simulink model "aerodynamic_model"  (R2021a)
settings: Solver=FixedStepAuto  StartTime=0  StopTime=10.0  FixedStep=T_sample_control  RelTol=1e-3  EnableMultiTasking=on
model workspace (MAT data in the model file):
  wing_alpha = 0.785398163397
libraries: vrlib x2
settings Model: DataDictionary=pid.sldd  EnableAccessToBaseWorkspace=off  ModifiedByFormat=The MathWorks Inc.  Creator=The MathWorks, Inc.  LastModifiedBy=The MathWorks Inc.
settings SolverCC: AlgebraicLoopSolver=TrustRegion
settings DataIOCC: SaveFormat=StructureWithTime  ReturnWorkspaceOutputs=off
settings OptimizationCC: BlockReduction=off  DefaultParameterBehavior=Inlined  InlineInvariantSignals=on  BufferReuse=off  PassReuseOutputArgsAs=Individual arguments  ExpressionDepthLimit=2147483647  ZeroExternalMemoryAtStartup=off  ZeroInternalMemoryAtStartup=off  EfficientFloat2IntCast=on  LifeSpan=1  EfficientTunableParamExpr=on
settings DebuggingCC: AlgebraicLoopMsg=none  FcnCallInpInsideContextMsg=warning  UnconnectedInputMsg=none  UnconnectedOutputMsg=none  UnconnectedLineMsg=none  UniqueDataStoreMsg=error  AssertControl=DisableAll  AllowSymbolicDim=off  StateNameClashWarn=warning  StrictBusMsg=ErrorOnBusTreatedAsVector  SFUnexpectedBacktrackingDiag=warning  SFNoUnconditionalDefaultTransitionDiag=warning  SFExecutionAtInitializationDiag=none  SFMachineParentedDataDiag=warning  ArithmeticOperatorsInVariantConditions=warning
settings HardwareCC: ProdBitPerPointer=32  ProdBitPerSizeT=32  ProdBitPerPtrDiffT=32  ProdLargestAtomicFloat=None  ProdIntDivRoundTo=Undefined  ProdEndianess=Unspecified  ProdWordSize=32  ProdHWDeviceType=32-bit Generic
settings ModelReferenceCC: PropagateSignalLabelsOutOfModel=off
settings SFSimCC: SimUseLocalCustomCode=off  CustomCodeUndefinedFunction=UseInterfaceOnly
settings RTWCC: SystemTargetFile=ert.tlc  TemplateMakefile=ert_default_tmf  GenerateReport=on  RTWUseLocalCustomCode=off  IncludeHyperlinkInReport=on  GenerateTraceInfo=on  GenerateTraceReport=on  GenerateTraceReportSl=on  GenerateTraceReportSf=on  GenerateTraceReportEml=on  GenerateCodeMetricsReport=on
settings CodeAppCC: IgnoreCustomStorageClasses=off  IgnoreTestpoints=on  CustomSymbolStrType=$N$R$M  StateflowObjectComments=on  InternalIdentifier=Classic
settings ERTTargetCC: MultiwordLength=2048  GenerateSampleERTMain=on  SupportNonFinite=off  ParenthesesLevel=Maximum  InlinedParameterPlacement=NonHierarchical  ERTCustomFileTemplate=example_file_process.tlc  ConvertIfToSwitch=off  SuppressUnreachableDefaultCases=off
settings ConfigComp: CovMetricSettings=dw  CovSaveCumulativeToWorkspaceVar=on  CovSaveSingleToWorkspaceVar=on  CovExternalEMLEnable=off  CovSFcnEnable=off

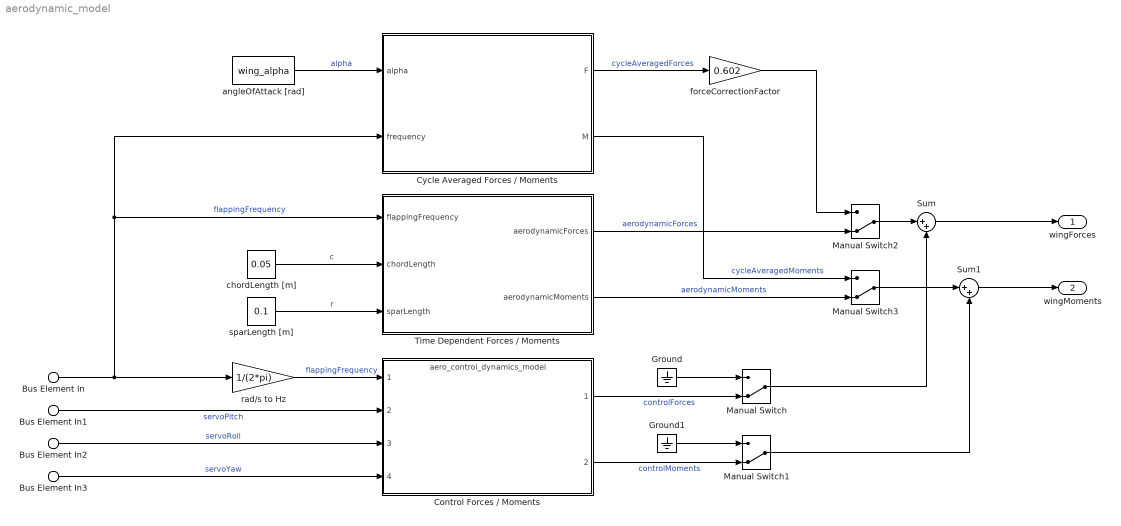
== system aerodynamic_model ==
  Bus Element In : Inport  PortName=flapFreq  Element=flapping_freq
  Bus Element In1 : Inport  PortName=flapFreq  Element=pitch
  Bus Element In2 : Inport  PortName=flapFreq  Element=roll
  Bus Element In3 : Inport  PortName=flapFreq  Element=yaw
  Control Forces / Moments : ModelReference  ModelNameDialog=aero_control_dynamics_model.slx  SimulationMode=Normal  ModelReferenceVersion=1.12
      mask Display: disp('Control Forces and Moments');
  Cycle Averaged Forces / Moments : MATLAB Function  TreatAsAtomicUnit=on
  Ground : Ground
  Ground1 : Ground
  Manual Switch{,1..3} (4 alike) : ManualSwitch  CurrentSetting=0
  Sum : Sum  Inputs=|++
  Sum1 : Sum  Inputs=|++
  Time Dependent Forces / Moments : Subsystem
      mask Display: disp('Time Dependent Forces and Moments');
  angleOfAttack [rad] : Constant  Value=wing_alpha
  chordLength [m] : Constant  Value=0.05
  forceCorrectionFactor : Gain  Gain=0.602
  rad/s to Hz : Gain  Gain=1/(2*pi)
  sparLength [m] : Constant  Value=0.1
  wingForces : Outport  PortDimensions=3
  wingMoments : Outport  Port=2  PortDimensions=3
  wires:
  Bus Element In1/1 -> Control Forces / Moments/2  "servoPitch"
  Bus Element In2/1 -> Control Forces / Moments/3  "servoRoll"
  Bus Element In3/1 -> Control Forces / Moments/4  "servoYaw"
  rad/s to Hz/1 -> Control Forces / Moments/1  "flappingFrequency"
  Sum/1 -> wingForces/1
  Sum1/1 -> wingMoments/1
  Control Forces / Moments/1 -> Manual Switch/2  "controlForces"
  Manual Switch/1 -> Sum/2
  Ground/1 -> Manual Switch/1
  Control Forces / Moments/2 -> Manual Switch1/2  "controlMoments"
  Ground1/1 -> Manual Switch1/1
  Manual Switch1/1 -> Sum1/2
  Bus Element In/1 -> Time Dependent Forces / Moments/1(flappingFrequency), Cycle Averaged Forces / Moments/2(frequency), rad/s to Hz/1  "flappingFrequency"
  angleOfAttack [rad]/1 -> Cycle Averaged Forces / Moments/1(alpha)  "alpha"
  Manual Switch2/1 -> Sum/1
  Cycle Averaged Forces / Moments/1(F) -> forceCorrectionFactor/1  "cycleAveragedForces"
  Manual Switch3/1 -> Sum1/1
  Cycle Averaged Forces / Moments/2(M) -> Manual Switch3/1  "cycleAveragedMoments"
  forceCorrectionFactor/1 -> Manual Switch2/1
  chordLength [m]/1 -> Time Dependent Forces / Moments/2(chordLength)  "c"
  sparLength [m]/1 -> Time Dependent Forces / Moments/3(sparLength)  "r"
  Time Dependent Forces / Moments/1(aerodynamicForces) -> Manual Switch2/2  "aerodynamicForces"
  Time Dependent Forces / Moments/2(aerodynamicMoments) -> Manual Switch3/2  "aerodynamicMoments"

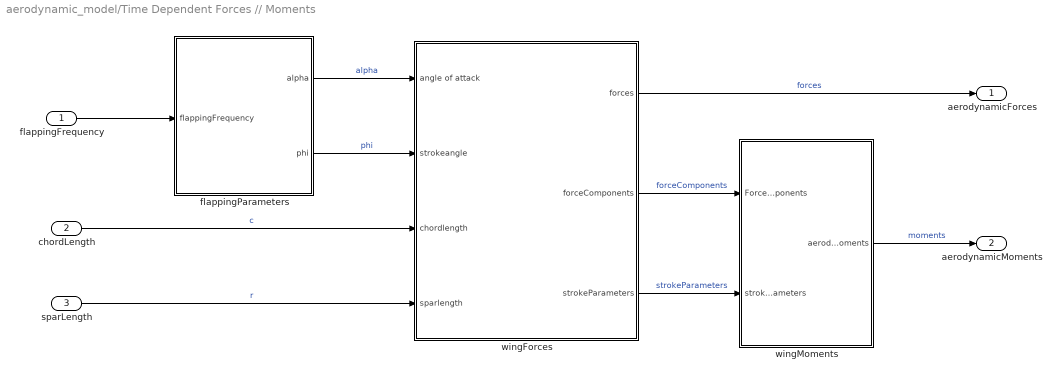
== system aerodynamic_model/Time Dependent Forces // Moments ==
  flappingFrequency : Inport
  chordLength : Inport  Port=2
  sparLength : Inport  Port=3
  flappingParameters : Subsystem
      mask Display: disp('Flapping Parameters');
  wingForces : Subsystem
      mask Display: disp('Wing Forces');
  wingMoments : Subsystem
      mask Display: disp('Wing Moments');
  aerodynamicForces : Outport
  aerodynamicMoments : Outport  Port=2
  wires:
  flappingParameters/1(alpha) -> wingForces/1(angle of attack)  "alpha"
  chordLength/1 -> wingForces/3(chordlength)  "c"
  flappingFrequency/1 -> flappingParameters/1(flappingFrequency)
  flappingParameters/2(phi) -> wingForces/2(strokeangle)  "phi"
  sparLength/1 -> wingForces/4(sparlength)  "r"
  wingMoments/1(aerodynamicMoments) -> aerodynamicMoments/1  "moments"
  wingForces/1(forces) -> aerodynamicForces/1  "forces"
  wingForces/3(strokeParameters) -> wingMoments/2(strokeParameters)  "strokeParameters"
  wingForces/2(forceComponents) -> wingMoments/1(ForceComponents)  "forceComponents"

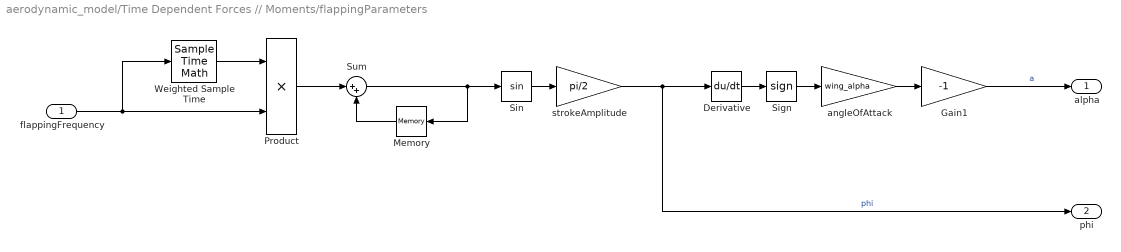
== system aerodynamic_model/Time Dependent Forces // Moments/flappingParameters ==
  flappingFrequency : Inport
  Derivative : Derivative
  Gain1 : Gain  Gain=-1
  Memory : Memory
  Product : Product
  Sign : Signum
  Sin : Trigonometry
  Sum : Sum  Inputs=|++
  Weighted Sample Time : SampleTimeMath  TsampMathOp=Ts Only
  angleOfAttack : Gain  Gain=wing_alpha
  strokeAmplitude : Gain  Gain=pi/2
  alpha : Outport
  phi : Outport  Port=2
  wires:
  Gain1/1 -> alpha/1  "a"
  flappingFrequency/1 -> Product/2, Weighted Sample Time/1
  Product/1 -> Sum/1
  Weighted Sample Time/1 -> Product/1
  Memory/1 -> Sum/2
  Sin/1 -> strokeAmplitude/1
  angleOfAttack/1 -> Gain1/1
  Sum/1 -> Sin/1, Memory/1
  Sign/1 -> angleOfAttack/1
  Derivative/1 -> Sign/1
  strokeAmplitude/1 -> Derivative/1, phi/1  "phi"

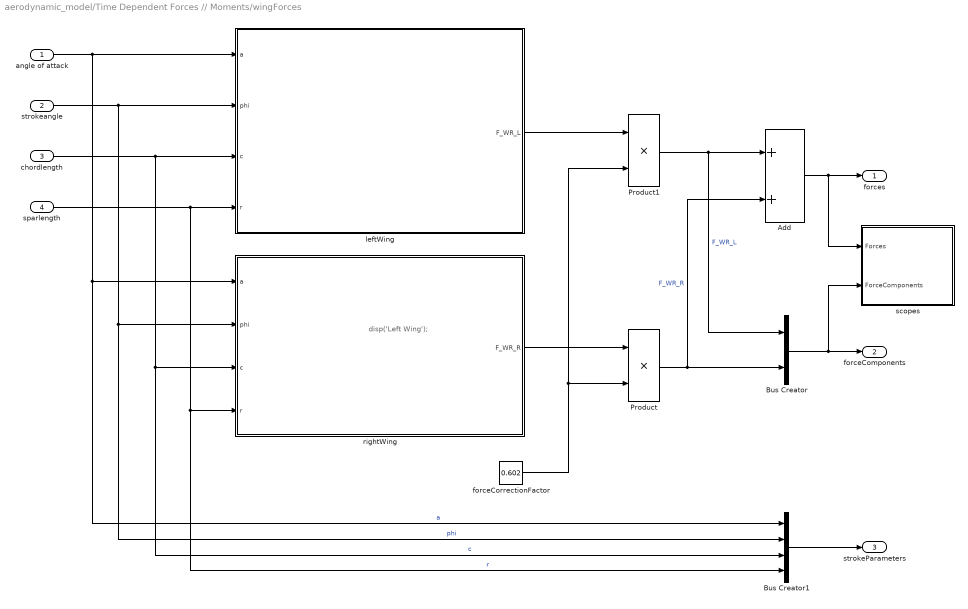
== system aerodynamic_model/Time Dependent Forces // Moments/wingForces ==
  note: disp('Left Wing');
  angle of attack : Inport
  strokeangle : Inport  Port=2
  chordlength : Inport  Port=3
  sparlength : Inport  Port=4
  Add : Sum
  Bus Creator : BusCreator  Inputs=2
  Bus Creator1 : BusCreator  Inputs=4
  Product : Product
  Product1 : Product
  forceCorrectionFactor : Constant  Value=0.602
  leftWing : Subsystem
      mask Display: disp('Left Wing');
  rightWing : Subsystem
      mask Display: disp('Right Wing');
  scopes : Subsystem
      mask Display: disp('Scopes');
  forces : Outport
  forceComponents : Outport  Port=2
  strokeParameters : Outport  Port=3
  wires:
  strokeangle/1 -> leftWing/2(phi), Bus Creator1/2, rightWing/2(phi)  "phi"
  angle of attack/1 -> Bus Creator1/1, rightWing/1(a), leftWing/1(a)  "a"
  Add/1 -> forces/1, scopes/1(Forces)
  chordlength/1 -> leftWing/3(c), Bus Creator1/3, rightWing/3(c)  "c"
  sparlength/1 -> leftWing/4(r), Bus Creator1/4, rightWing/4(r)  "r"
  Bus Creator/1 -> scopes/2(ForceComponents), forceComponents/1
  Product1/1 -> Add/1, Bus Creator/1  "F_WR_L"
  Product/1 -> Bus Creator/2, Add/2  "F_WR_R"
  leftWing/1(F_WR_L) -> Product1/1
  rightWing/1(F_WR_R) -> Product/1
  forceCorrectionFactor/1 -> Product1/2, Product/2
  Bus Creator1/1 -> strokeParameters/1

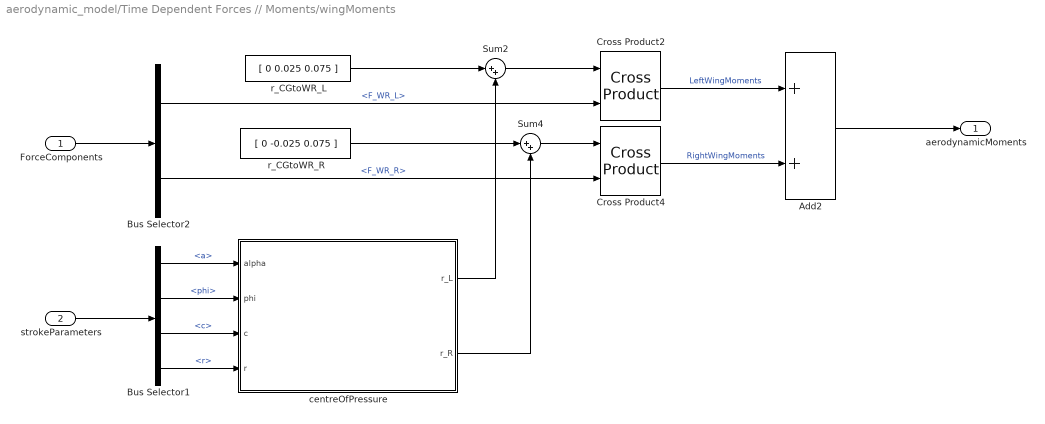
== system aerodynamic_model/Time Dependent Forces // Moments/wingMoments ==
  ForceComponents : Inport
  strokeParameters : Inport  Port=2
  Add2 : Sum
  Bus Selector1 : BusSelector  OutputSignals=a,phi,c,r
  Bus Selector2 : BusSelector  OutputSignals=F_WR_L,F_WR_R
  Cross Product2 : vrlib/Utilities/Cross Product
  Cross Product4 : vrlib/Utilities/Cross Product
  Sum2 : Sum  Inputs=|++
  Sum4 : Sum  Inputs=|++
  centreOfPressure : MATLAB Function  TreatAsAtomicUnit=on
  r_CGtoWR_L : Constant  Value=[ 0 0.025 0.075 ]
  r_CGtoWR_R : Constant  Value=[ 0 -0.025 0.075 ]
  aerodynamicMoments : Outport
  wires:
  strokeParameters/1 -> Bus Selector1/1
  Bus Selector1/1 -> centreOfPressure/1(alpha)  "<a>"
  Bus Selector1/2 -> centreOfPressure/2(phi)  "<phi>"
  Bus Selector1/3 -> centreOfPressure/3(c)  "<c>"
  Bus Selector1/4 -> centreOfPressure/4(r)  "<r>"
  Add2/1 -> aerodynamicMoments/1
  Bus Selector2/1 -> Cross Product2/2  "<F_WR_L>"
  ForceComponents/1 -> Bus Selector2/1
  r_CGtoWR_R/1 -> Sum4/1
  Sum4/1 -> Cross Product4/1
  Cross Product4/1 -> Add2/2  "RightWingMoments"
  centreOfPressure/1(r_L) -> Sum2/2
  Bus Selector2/2 -> Cross Product4/2  "<F_WR_R>"
  r_CGtoWR_L/1 -> Sum2/1
  Sum2/1 -> Cross Product2/1
  centreOfPressure/2(r_R) -> Sum4/2
  Cross Product2/1 -> Add2/1  "LeftWingMoments"

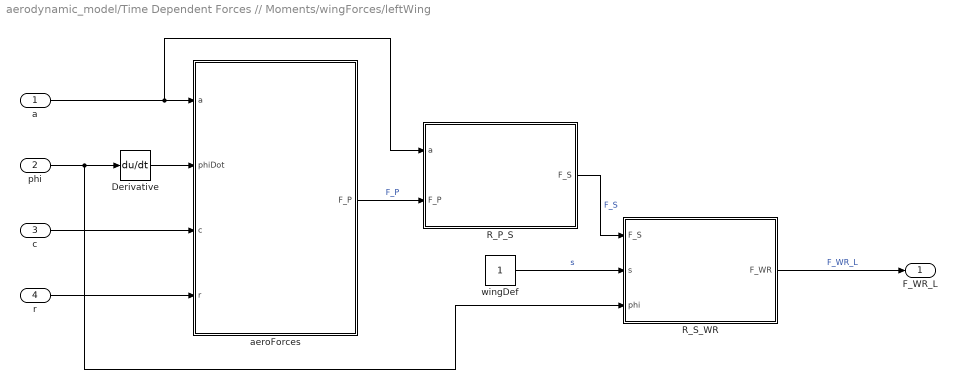
== system aerodynamic_model/Time Dependent Forces // Moments/wingForces/leftWing ==
  a : Inport
  phi : Inport  Port=2
  c : Inport  Port=3
  r : Inport  Port=4
  Derivative : Derivative
  R_P_S : MATLAB Function  TreatAsAtomicUnit=on
  R_S_WR : MATLAB Function  TreatAsAtomicUnit=on
  aeroForces : MATLAB Function  TreatAsAtomicUnit=on
  wingDef : Constant
  F_WR_L : Outport
  wires:
  a/1 -> R_P_S/1(a), aeroForces/1(a)
  c/1 -> aeroForces/3(c)
  aeroForces/1(F_P) -> R_P_S/2(F_P)  "F_P"
  R_P_S/1(F_S) -> R_S_WR/1(F_S)  "F_S"
  wingDef/1 -> R_S_WR/2(s)  "s"
  phi/1 -> R_S_WR/3(phi), Derivative/1
  r/1 -> aeroForces/4(r)
  Derivative/1 -> aeroForces/2(phiDot)
  R_S_WR/1(F_WR) -> F_WR_L/1  "F_WR_L"

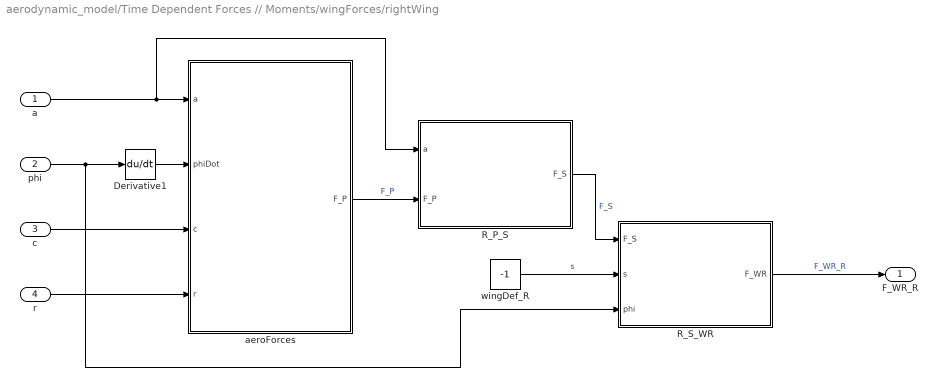
== system aerodynamic_model/Time Dependent Forces // Moments/wingForces/rightWing ==
  a : Inport
  phi : Inport  Port=2
  c : Inport  Port=3
  r : Inport  Port=4
  Derivative1 : Derivative
  R_P_S : MATLAB Function  TreatAsAtomicUnit=on
  R_S_WR : MATLAB Function  TreatAsAtomicUnit=on
  aeroForces : MATLAB Function  TreatAsAtomicUnit=on
  wingDef_R : Constant  Value=-1
  F_WR_R : Outport
  wires:
  aeroForces/1(F_P) -> R_P_S/2(F_P)  "F_P"
  Derivative1/1 -> aeroForces/2(phiDot)
  c/1 -> aeroForces/3(c)
  wingDef_R/1 -> R_S_WR/2(s)  "s"
  R_S_WR/1(F_WR) -> F_WR_R/1  "F_WR_R"
  a/1 -> R_P_S/1(a), aeroForces/1(a)
  R_P_S/1(F_S) -> R_S_WR/1(F_S)  "F_S"
  r/1 -> aeroForces/4(r)
  phi/1 -> R_S_WR/3(phi), Derivative1/1

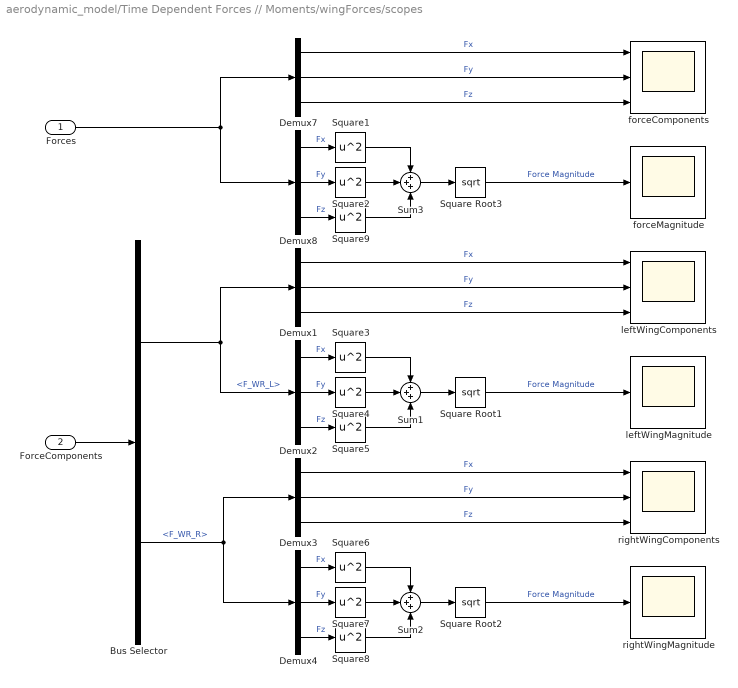
== system aerodynamic_model/Time Dependent Forces // Moments/wingForces/scopes ==
  Forces : Inport
  ForceComponents : Inport  Port=2
  Bus Selector : BusSelector  OutputSignals=F_WR_L,F_WR_R
  Demux{1..4,7..8} (6 alike) : Demux  Outputs=3
  Square Root1 : Sqrt  SaturateOnIntegerOverflow=on
  Square Root2 : Sqrt  SaturateOnIntegerOverflow=on
  Square Root3 : Sqrt  SaturateOnIntegerOverflow=on
  Square{1..9} (9 alike) : Math  Operator=square  SaturateOnIntegerOverflow=on
  Sum1 : Sum  Inputs=+++
  Sum2 : Sum  Inputs=+++
  Sum3 : Sum  Inputs=+++
  forceComponents : Scope  NumInputPorts=3
  forceMagnitude : Scope
  leftWingComponents : Scope  NumInputPorts=3
  leftWingMagnitude : Scope
  rightWingComponents : Scope  NumInputPorts=3
  rightWingMagnitude : Scope
  wires:
  Forces/1 -> Demux8/1, Demux7/1
  Demux8/3 -> Square9/1  "Fz"
  Square Root3/1 -> forceMagnitude/1  "Force Magnitude"
  Square1/1 -> Sum3/1
  Square2/1 -> Sum3/2
  Demux7/1 -> forceComponents/1  "Fx"
  Demux7/2 -> forceComponents/2  "Fy"
  Demux7/3 -> forceComponents/3  "Fz"
  Demux8/2 -> Square2/1  "Fy"
  Demux8/1 -> Square1/1  "Fx"
  Sum3/1 -> Square Root3/1
  Square9/1 -> Sum3/3
  Square5/1 -> Sum1/3
  Sum1/1 -> Square Root1/1
  Demux2/1 -> Square3/1  "Fx"
  Demux2/2 -> Square4/1  "Fy"
  Demux1/3 -> leftWingComponents/3  "Fz"
  Demux1/2 -> leftWingComponents/2  "Fy"
  Demux1/1 -> leftWingComponents/1  "Fx"
  Square4/1 -> Sum1/2
  Square3/1 -> Sum1/1
  Square Root1/1 -> leftWingMagnitude/1  "Force Magnitude"
  Demux2/3 -> Square5/1  "Fz"
  ForceComponents/1 -> Bus Selector/1
  Bus Selector/1 -> Demux2/1, Demux1/1  "<F_WR_L>"
  Demux4/3 -> Square8/1  "Fz"
  Square Root2/1 -> rightWingMagnitude/1  "Force Magnitude"
  Square6/1 -> Sum2/1
  Square7/1 -> Sum2/2
  Demux3/1 -> rightWingComponents/1  "Fx"
  Demux3/2 -> rightWingComponents/2  "Fy"
  Demux3/3 -> rightWingComponents/3  "Fz"
  Demux4/2 -> Square7/1  "Fy"
  Demux4/1 -> Square6/1  "Fx"
  Sum2/1 -> Square Root2/1
  Square8/1 -> Sum2/3
  Bus Selector/2 -> Demux4/1, Demux3/1  "<F_WR_R>"

== matlab function aerodynamic_model/Time Dependent Forces // Moments/wingForces/leftWing/R_S_WR ==
  data: F_S input; s input; phi input; F_WR output
function F_WR = S_to_WR(F_S,s,phi)

arg = s*phi;

R_S_WR = [  
           cos(arg)  -sin(arg)    0 ;
           sin(arg)   cos(arg)    0 ;
              0          0        1 ;
         ];

F_WR = R_S_WR * F_S;

end

== matlab function aerodynamic_model/Time Dependent Forces // Moments/wingForces/leftWing/aeroForces ==
  data: a input; F_P output; phiDot input; c input; r input
function F_P = aeroForces(a,phiDot,c,r)

% Declare sizes
F_P = zeros(3,1);

% Define the density of air [kg/m^3]
p = 1.225; 

% Define the value of the F-P angle theta
theta = -a;

% Define the lift and drag coefficients using the absolute value of alpha
cL = 0.225 + 1.58*sin((2.13*abs(a))-(7.2*(pi()/180)));
cD = 1.92 - 1.55*cos((2.04*abs(a))-(9.82*(pi()/180)));

% Calculate the cartesian components of the force vector in the P frame
Fx_P = (-1/6)*cos(theta)*sign(a)*p*(phiDot^2)*cD*c*(r^3) + (1/6)*sin(theta)*p*(phiDot^2)*cL*c*(r^3);
Fy_P = 0;
Fz_P = (1/6)*sin(theta)*sign(a)*p*(phiDot^2)*cD*c*(r^3) + (1/6)*cos(theta)*p*(phiDot^2)*cL*c*(r^3);

% Construct the force vector in the P frame
F_P = [ Fx_P ;
        Fy_P ; 
        Fz_P ; ];

end

== matlab function aerodynamic_model/Time Dependent Forces // Moments/wingForces/leftWing/R_P_S ==
  data: a input; F_P input; F_S output
function F_S = P_to_S(a,F_P)

R_P_S = [  
           cos(a)   0   sin(a) ;
             0      1     0    ;
          -sin(a)   0   cos(a) ;
        ];

F_S = R_P_S * F_P;

end

== matlab function aerodynamic_model/Time Dependent Forces // Moments/wingForces/rightWing/R_P_S ==
  data: a input; F_P input; F_S output
function F_S = P_to_S(a,F_P)

R_P_S = [  
           cos(a)   0   sin(a) ;
             0      1     0    ;
          -sin(a)   0   cos(a) ;
        ];

F_S = R_P_S * F_P;

end

== matlab function aerodynamic_model/Time Dependent Forces // Moments/wingForces/rightWing/R_S_WR ==
  data: F_S input; s input; phi input; F_WR output
function F_WR = S_to_WR(F_S,s,phi)

arg = s*phi;

R_S_WR = [  
           cos(arg)  -sin(arg)    0 ;
           sin(arg)   cos(arg)    0 ;
              0          0        1 ;
         ];

F_WR = R_S_WR * F_S;

end

== matlab function aerodynamic_model/Time Dependent Forces // Moments/wingForces/rightWing/aeroForces ==
  data: a input; F_P output; phiDot input; c input; r input
function F_P = aeroForces(a,phiDot,c,r)

% Declare sizes
F_P = zeros(3,1);

% Define the density of air [kg/m^3]
p = 1.225; 

% Define the value of the F-P angle theta
theta = -a;

% Define the lift and drag coefficients using the absolute value of alpha
cL = 0.225 + 1.58*sin((2.13*abs(a))-(7.2*(pi()/180)));
cD = 1.92 - 1.55*cos((2.04*abs(a))-(9.82*(pi()/180)));

% Calculate the cartesian components of the force vector in the P frame
Fx_P = (-1/6)*cos(theta)*sign(a)*p*(phiDot^2)*cD*c*(r^3) + (1/6)*sin(theta)*p*(phiDot^2)*cL*c*(r^3);
Fy_P = 0;
Fz_P = (1/6)*sin(theta)*sign(a)*p*(phiDot^2)*cD*c*(r^3) + (1/6)*cos(theta)*p*(phiDot^2)*cL*c*(r^3);

% Construct the force vector in the P frame
F_P = [ Fx_P ;
        Fy_P ; 
        Fz_P ; ];

end

== matlab function aerodynamic_model/Cycle Averaged Forces // Moments ==
  data: alpha input; F output; frequency input; M output
function [F,M] = cycleAveraging(alpha, frequency)
if frequency > 0
    F = real(cycleAveragedForce(alpha, frequency, frequency));
    M = real(cycleAveragedMoment(alpha, frequency, frequency));
else
    F = [0,0,0];
    M = [0,0,0];

end

== matlab function aerodynamic_model/Time Dependent Forces // Moments/wingMoments/centreOfPressure ==
  data: alpha input; r_L output; phi input; c input; r input; r_R output
function [r_L,r_R] = r_CP(alpha,phi,c,r)

r_L = zeros(3,1);
r_R = zeros(3,1);

% This function generates the distance to the centre of pressure for each
% wing in the wing root frame. This distance is then added to the CG to WR
% distance for each wing to generate the total moment arm. 
%
% The definition of centre of pressure used here is arbitrarily set to be
% the midpoint of the wing. This is an assumption that is expected to be
% improved moving forward, with this script serving as a baseline for
% future work. See the Maple file for more infomation about this
% derivation.

% Left Wing

s = 1;

r_L = [  (1/2)*cos(s*phi)*sin(alpha)*c + (1/2)*sin(s*phi)*s*r ;
        -(1/2)*sin(s*phi)*sin(alpha)*c + (1/2)*cos(s*phi)*s*r ; 
                               -(1/2)*cos(alpha)*c            ;
      ];      

% Right Wing

s = -1;

r_R = [  (1/2)*cos(s*phi)*sin(alpha)*c + (1/2)*sin(s*phi)*s*r ;
        -(1/2)*sin(s*phi)*sin(alpha)*c + (1/2)*cos(s*phi)*s*r ; 
                               -(1/2)*cos(alpha)*c            ;
      ];
      
end
